simulink model "sepicmm"  (R2015a)
settings: Solver=ode45  StartTime=0.0  StopTime=1  RelTol=1e-3
values from neighbouring files (symbols this model uses):
  alpha = min(d1,d2)    [Final_2.m]    (also in Final_discreto.m)
  Ao = Aaum-L*Caum    [Final_2.m]
  Bo = [Baum L]    [Final_2.m]
  C = [0 0 0 1]    [Final_2.m]    (also in Final_discreto.m)
  C1 = 190e-6    (= 0.00019)    [Final_2.m]    (also in Final_discreto.m = 0.0022)
  C2 = 190e-6    (= 0.00019)    [Final_2.m]    (also in Final_discreto.m = 0.0022)
  Co = [eye(size(Ao,1)-1) zeros(size(Ao,1)-1,1)]    [Final_2.m]
  Do = zeros(size(Ao,1)-1,2)    [Final_2.m]
  E0 = 20    [Final_2.m]    (also in Final_discreto.m = 36)
  ki = Ki_(5,1)    [Final_2.m]
  ks = [Ki_(1,1) Ki_(2,1) Ki_(3,1) Ki_(4,1) ]'    [Final_2.m]
  L = L'    [Final_2.m]
  L1 = 2.3e-3    (= 0.0023)    [Final_2.m]    (also in Final_discreto.m = 0.00156)
  L2 = 330e-6    (= 0.00033)    [Final_2.m]    (also in Final_discreto.m = 0.00324)
  R0 = 44    [Final_2.m]    (also in Final_discreto.m = 50)
  R1 = 2.134    [Final_2.m]    (also in Final_discreto.m = 0.3)
  R2 = 0.234    [Final_2.m]    (also in Final_discreto.m = 0.3)
  V0 = 20    [Final_2.m]    (also in Final_discreto.m = 120)
undefined symbols (not defined in the file or in its folder): Rl
libraries: powerlib x17
settings Model: CovSFcnEnable=off  Creator=estudiante  LastModifiedBy=berme_000
settings DebuggingCC: SolverPrmCheckMsg=warning

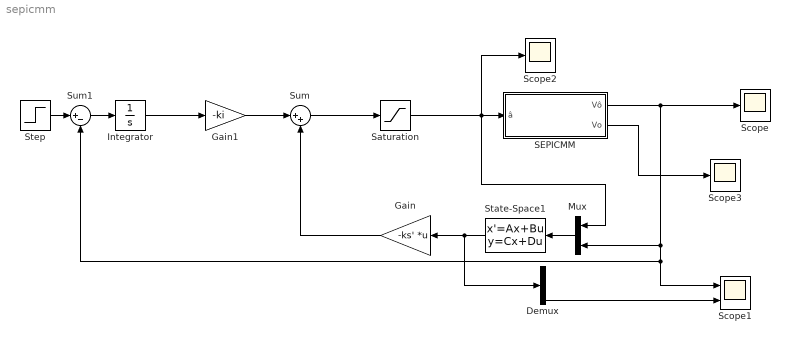
== system sepicmm ==
  Demux : Demux
  Gain : Gain  Gain=-ks'  Multiplication=Matrix(K*u)
  Gain1 : Gain  Gain=-ki
  Integrator : Integrator
  Mux : Mux  Inputs=2
  "SEPICMM " : Subsystem
  Saturation : Saturate  UpperLimit=1-alpha  LowerLimit=0.5-alpha
  Scope : Scope
      settings: YMin=-4.25e-09  YMax=-2.5e-10
  Scope1 : Scope  NumInputPorts=2
      settings: YMin=-120~-119.98  YMax=-120~-119.86
  Scope2 : Scope
      settings: YMin=0.216701  YMax=0.216701  SaveName=ScopeData3
  Scope3 : Scope
      settings: TimeRange=1  YMin=75  YMax=140  SaveName=ScopeData4
  State-Space1 : StateSpace  A=Ao  B=Bo  C=Co  D=Do  X0=0
  Step : Step  Time=0.5  After=45  SampleTime=0
  Sum : Sum  Inputs=|++
  Sum1 : Sum  Inputs=|+-
  wires:
  Mux/1 -> State-Space1/1
  State-Space1/1 -> Demux/1, Gain/1
  Integrator/1 -> Gain1/1
  Gain1/1 -> Sum/1
  Gain/1 -> Sum/2
  Demux/4 -> Scope1/2
  "SEPICMM "/2(Vo) -> Scope3/1
  Saturation/1 -> "SEPICMM "/1(â), Scope2/1, Mux/1
  "SEPICMM "/1(Vô) -> Sum1/2, Scope1/1, Mux/2, Scope/1
  Step/1 -> Sum1/1
  Sum1/1 -> Integrator/1
  Sum/1 -> Saturation/1

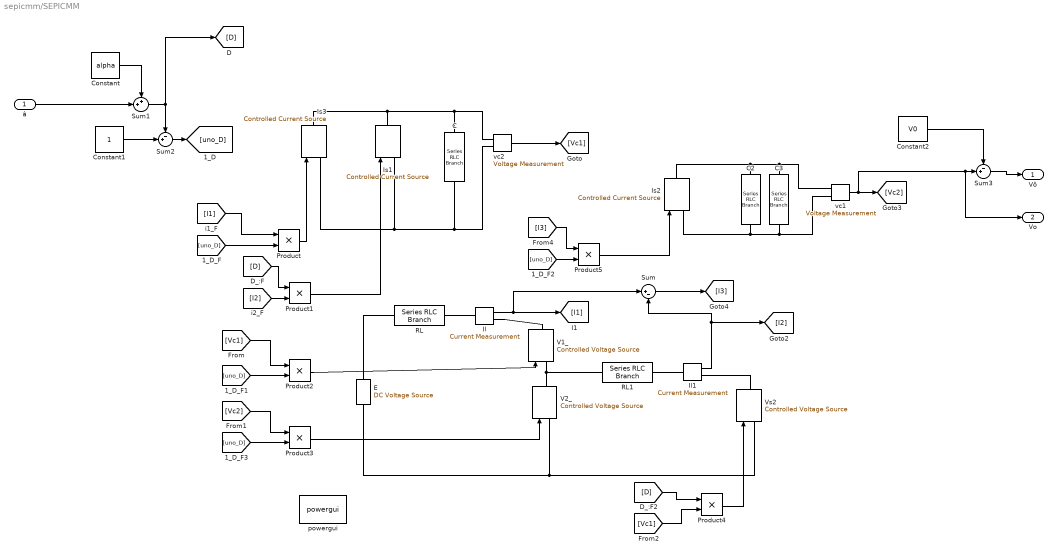
== system sepicmm/SEPICMM  ==
  â : Inport
  C : powerlib/Elements/Series RLC Branch  LConnTagsString=__new0  RConnTagsString=__new0  BranchType=C  Resistance=Rl  Inductance=L  SetiL0=off  InitialCurrent=0  Capacitance=C1  Setx0=on  InitialVoltage=Vc1  Measurements=None
  C2 : powerlib/Elements/Series RLC Branch  LConnTagsString=__new0  RConnTagsString=__new0  BranchType=C  Resistance=Rl  Inductance=L  SetiL0=off  InitialCurrent=0  Capacitance=C2  Setx0=on  InitialVoltage=V0  Measurements=None
  C3 : powerlib/Elements/Series RLC Branch  LConnTagsString=__new0  RConnTagsString=__new0  BranchType=R  Resistance=R0  Inductance=L  SetiL0=off  InitialCurrent=0  Capacitance=C  Setx0=off  InitialVoltage=0  Measurements=None
  Constant : Constant  Value=alpha
  Constant1 : Constant
  Constant2 : Constant  Value=V0
  E : powerlib/Electrical Sources/DC Voltage Source  Amplitude=E0  Measurements=Voltage
  Il : powerlib/Measurements/Current Measurement  PhasorSimulation=off  OutputType=Complex  PSBequivalent=0
  Il1 : powerlib/Measurements/Current Measurement  PhasorSimulation=off  OutputType=Complex  PSBequivalent=0
  Is1 : powerlib/Electrical Sources/Controlled Current Source  Initialize=on  Source_Type=AC  Amplitude=0  Phase=0  Frequency=0  Measurements=None
  Is2 : powerlib/Electrical Sources/Controlled Current Source  Initialize=on  Source_Type=AC  Amplitude=0  Phase=0  Frequency=0  Measurements=None
  Is3 : powerlib/Electrical Sources/Controlled Current Source  Initialize=on  Source_Type=AC  Amplitude=0  Phase=0  Frequency=0  Measurements=None
  Product{,1..5} (6 alike) : Product
  RL : powerlib/Elements/Series RLC Branch  LConnTagsString=__new0  RConnTagsString=__new0  BranchType=RL  Resistance=R1  Inductance=L1  SetiL0=on  InitialCurrent=il1  Capacitance=1e-6  Setx0=off  InitialVoltage=0  Measurements=None
  RL1 : powerlib/Elements/Series RLC Branch  LConnTagsString=__new0  RConnTagsString=__new0  BranchType=RL  Resistance=R2  Inductance=L2  SetiL0=on  InitialCurrent=il2  Capacitance=1e-6  Setx0=off  InitialVoltage=0  Measurements=None
  Sum : Sum  Inputs=|+-
  Sum1 : Sum  Inputs=++|
  Sum2 : Sum  Inputs=-+|
  Sum3 : Sum  Inputs=-+|
  V1_ : powerlib/Electrical Sources/Controlled Voltage Source  Initialize=on  Source_Type=AC  Amplitude=0  Phase=0  Frequency=0  Measurements=None
  V2_ : powerlib/Electrical Sources/Controlled Voltage Source  Initialize=on  Source_Type=AC  Amplitude=0  Phase=0  Frequency=0  Measurements=None
  Vs2 : powerlib/Electrical Sources/Controlled Voltage Source  Initialize=on  Source_Type=AC  Amplitude=0  Phase=0  Frequency=0  Measurements=None
  powergui : powerlib/powergui  Priority=1  SimulationMode=Continuous  SolverType=Tustin  SampleTime=50e-6  frequency=60  SPID=off  DisableSnubberDevices=off  DisableRonSwitches=off  DisableVfSwitches=off  SwTol=0  DisplayEquations=off  Interpol=off  methode=off  Ts=0  FunctionMessages=off  echomessages=off  HookPort=off  EnableUseOfTLC=off  x0status=blocks  frequencyindice=0  Pbase=100e6  ErrMax=1e-4  Iterations=50  UnitsV=kV  UnitsW=MW  buscounter=0  RestoreLinks=warning  ResistiveCurrentMeasurement=off  Frange=[0:2:500]  Ylog=off  Xlog=on  ShowGrid=off  save=off  variable=ZData  structure=0  ZoomFFT=off  StartTime=0.0  cycles=1  DisplayStyle=1  fundamental=60  FreqAxis=off  MaxFrequency=1000  frequencyindicesteady=1  RmsSteady=1  display=off
  vc1 : powerlib/Measurements/Voltage Measurement  PhasorSimulation=off  OutputType=Complex  PSBequivalent=0
  vc2 : powerlib/Measurements/Voltage Measurement  PhasorSimulation=off  OutputType=Complex  PSBequivalent=0
  Vô : Outport
  Vo : Outport  Port=2
  wires:
  Il/1 -> Sum/1, [I1]
  Il1/1 -> [I2], Sum/2
  vc2/1 -> [Vc1]
  Sum/1 -> [I3]
  Sum1/1 -> [D], Sum2/1
  Constant/1 -> Sum1/1
  Constant1/1 -> Sum2/2
  Constant2/1 -> Sum3/1
  vc1/1 -> Vo/1, Sum3/2, [Vc2]
  Sum3/1 -> Vô/1
  [I1] -> Product/1
  Product/1 -> Is3/1
  [uno_D] -> Product/2
  [I2] -> Product1/2
  [D] -> Product1/1
  Product1/1 -> Is1/1
  [uno_D] -> Product2/2
  [Vc1] -> Product2/1
  Product2/1 -> V1_/1
  [Vc2] -> Product3/1
  [uno_D] -> Product3/2
  Product3/1 -> V2_/1
  Product4/1 -> Vs2/1
  [Vc1] -> Product4/2
  [uno_D] -> Product5/2
  [I3] -> Product5/1
  Product5/1 -> Is2/1
  Sum2/1 -> [uno_D]
  â/1 -> Sum1/2
  [D] -> Product4/1
  connections:
  V1_/LConn1 -- RL1/LConn1 -- V2_/RConn1
  V2_/LConn1 -- Vs2/LConn1 -- E/LConn1
  Is3/LConn1 -- Is1/LConn1 -- vc2/LConn2 -- C/RConn1
  C2/LConn1 -- Is2/RConn1 -- vc1/LConn1 -- C3/LConn1
  Is2/LConn1 -- C2/RConn1 -- vc1/LConn2 -- C3/RConn1
  C/LConn1 -- vc2/LConn1 -- Is3/RConn1 -- Is1/RConn1
  Il/RConn1 -- V1_/RConn1
  RL/LConn1 -- E/RConn1
  Il/LConn1 -- RL/RConn1
  Il1/LConn1 -- RL1/RConn1
  Il1/RConn1 -- Vs2/RConn1
